simulink model "window_stateflow"  (R2025a)
settings: Solver=VariableStepAuto  StartTime=0.0  StopTime=10.0  RelTol=1e-3
settings Model: Creator=ISI  LastModifiedBy=ISI

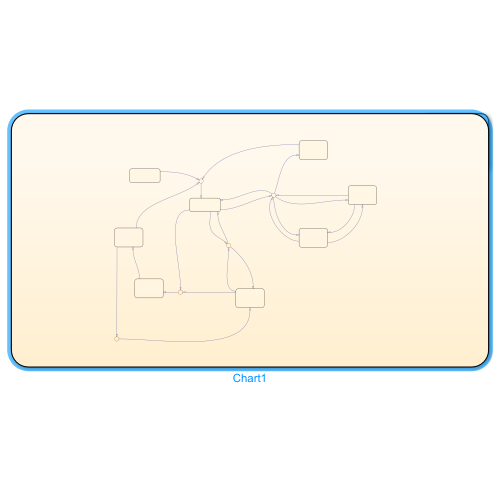
[thumbnail: Simulink's stored preview of the top-level diagram]
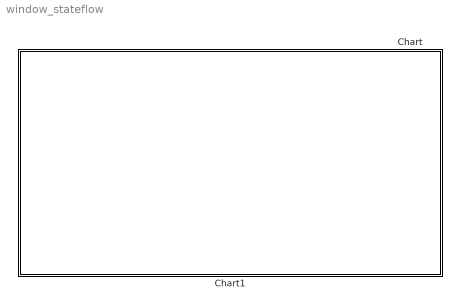
== system window_stateflow ==
  Chart : Stateflow chart  TreatAsAtomicUnit=on
  Chart1 : Stateflow chart  TreatAsAtomicUnit=on

== stateflow chart window_stateflow/Chart ==

== stateflow chart window_stateflow/Chart1 ==
  state Config
  state Init
  state Eph_Input
  state Standby
  state Waking_up
  state Manual
  state Sleep
  state Auto_Mode
  Config -> (junction 70) : [end_submit]
  (junction 41) -> Config [order 2] : [begin_config]
  Init -> (junction 70) : [1]
  Waking_up -> (junction 70) [order 1] : [auto_mode = 0 && data_loaded = 1]
  (junction 70) -> Standby
  (junction 41) -> Standby [order 1]
  Eph_Input -> (junction 41) [order 1] : [end_eph_input]
  Standby -> (junction 41) [order 2]
  (junction 41) -> Eph_Input [order 3] : [begin_eph_input]
  Manual -> (junction 41) [order 1] : [end_manual]
  (junction 41) -> Manual [order 4] : [begin_manual]
  Eph_Input -> Manual [order 2] : [begin_manual]
  Manual -> Eph_Input [order 2] : [begin_eph_input]
  Standby -> (junction 74) [order 1]
  Standby -> (junction 83) [order 3] : [toggle_auto_mode]
  (junction 83) -> Standby [order 1] : [auto_mode = 1]
  (junction 83) -> Auto_Mode [order 2] : [auto_mode = 0]
  Waking_up -> (junction 89) [order 2]
  Sleep -> Waking_up : [wake_up]
  Auto_Mode -> (junction 83) [order 2] : [toggle_auto_mode]
  (junction 74) -> Sleep : [go_sleep]
  Auto_Mode -> (junction 74) [order 1]
  (junction 89) -> Auto_Mode : [[auto_mode = 0 && data_loaded = 1]]
